simulink library "libAggregators"  (R2015a)
settings: Solver=ode45  StartTime=0.0  StopTime=10.0  RelTol=1e-3
libraries: dspsigattribs x4, libAggregators x1
settings Model: Creator=jcardena  LastModifiedBy=jcardena
settings DebuggingCC: UnderspecifiedInitializationDetection=Classic  MergeDetectMultiDrivingBlocksExec=none  SolverPrmCheckMsg=warning  StateNameClashWarn=warning

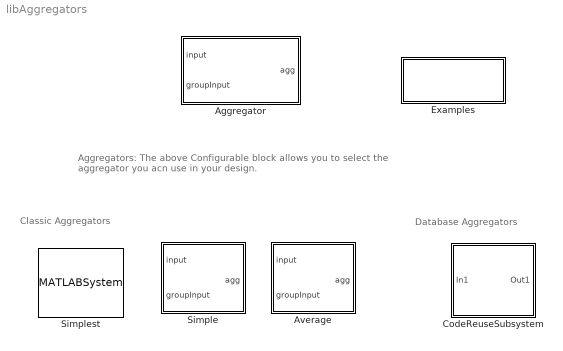
== system libAggregators ==
  note: Aggregators: The above Configurable block allows you to select the aggregator you acn use in your design.
  note: Database Aggregators
  note: Classic Aggregators
  Aggregator : Subsystem  BlockChoice=Average
      settings: TemplateBlock=self  MemberBlocks=Average,Simple
  Average : Subsystem  mask(aggregatingBlock){gVal=1}
      mask prompts: gVal "Grouping expression or value"
      mask help: An Aggregator classifies data rows from a single input link into groups and computes totals or other aggregate functions for each group. The averaged totals for each group are output from the stage via an output port.
      settings: RTWFcnNameOpts=Use subsystem name  RTWFileNameOpts=Use function name
      mask Help: Enter the aggregate function
      mask Display: image('images/aggrIcon.png')
  CodeReuseSubsystem : Subsystem  TreatAsAtomicUnit=on  mask(Aggregator Type){}
      mask help: Aggregator description
      settings: RTWFcnNameOpts=Use subsystem name  RTWFileNameOpts=Use function name
  Examples : Subsystem  mask(Aggregator Examples){}
      mask Display: disp('Aggregator\nExamples')
  Simple : Subsystem  mask(aggregatingBlock){gVal=1}
      mask prompts: gVal "Grouping expression or value"
      mask help: An Aggregator classifies data rows from a single input link into groups and computes totals or other aggregate functions for each group. The summed totals for each group are output from the stage via an output port.
      mask Help: Enter the aggregate function
      mask Display: image('images/aggrIcon.png')
  Simplest : MATLABSystem  System=simplestAggregator_mtlbSysBlock
      mask Type: simplestAggregator_mtlbSysBlock
      mask Display:
      | disp('Simplest');
      | port_label('output',1,'agg');

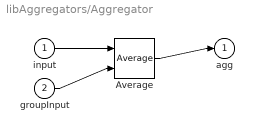
== system libAggregators/Aggregator ==
  input : Inport
  groupInput : Inport  Port=2
  Average : libAggregators/Average  gVal=1
  agg : Outport
  wires:
  input/1 -> Average/1
  groupInput/1 -> Average/2
  Average/1 -> agg/1

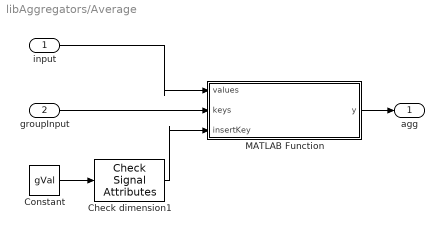
== system libAggregators/Average ==
  input : Inport
  groupInput : Inport  Port=2
  Check dimension1 : dspsigattribs/Check Signal Attributes  SigAttribCheckMethod=Does not match attributes exactly  Complexity=Ignore  Frame=Ignore  DimsCheckMethod=Is...  Dimensions=Vector (1-D or 2-D)  DatatypeCheckMethod=Ignore  DatatypeGeneral=Floating-point  DtypeFloatSpecific=Any floating-point  DtypeFixedSpecific=Any fixed-point  DtypeIntSpecific=Any integer  SampleMode=Ignore
  Constant : Constant  Value=gVal
  MATLAB Function : MATLAB Function  TreatAsAtomicUnit=on
      settings: RTWSystemCode=Inline
  agg : Outport
  wires:
  input/1 -> MATLAB Function/1(values)
  groupInput/1 -> MATLAB Function/2(keys)
  Constant/1 -> Check dimension1/1
  MATLAB Function/1(y) -> agg/1
  Check dimension1/1 -> MATLAB Function/3(insertKey)

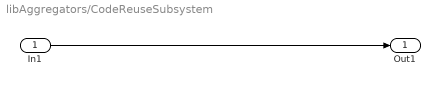
== system libAggregators/CodeReuseSubsystem ==
  In1 : Inport
  Out1 : Outport
  wires:
  In1/1 -> Out1/1

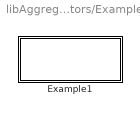
== system libAggregators/Examples ==
  Example1 : Subsystem
      settings: OpenFcn=read_simulated_unitIDs_example

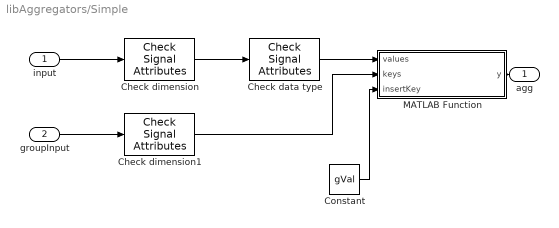
== system libAggregators/Simple ==
  input : Inport
  groupInput : Inport  Port=2
  Check data type : dspsigattribs/Check Signal Attributes  SigAttribCheckMethod=Does not match attributes exactly  Complexity=Ignore  Frame=Ignore  DimsCheckMethod=Ignore  Dimensions=Full matrix (2-D)  DatatypeCheckMethod=Is...  DatatypeGeneral=Floating-point  DtypeFloatSpecific=Double precision  DtypeFixedSpecific=Any fixed-point  DtypeIntSpecific=Any integer  SampleMode=Ignore
  Check dimension : dspsigattribs/Check Signal Attributes  SigAttribCheckMethod=Does not match attributes exactly  Complexity=Ignore  Frame=Ignore  DimsCheckMethod=Is...  Dimensions=Vector (1-D or 2-D)  DatatypeCheckMethod=Ignore  DatatypeGeneral=Floating-point  DtypeFloatSpecific=Any floating-point  DtypeFixedSpecific=Any fixed-point  DtypeIntSpecific=Any integer  SampleMode=Ignore
  Check dimension1 : dspsigattribs/Check Signal Attributes  SigAttribCheckMethod=Does not match attributes exactly  Complexity=Ignore  Frame=Ignore  DimsCheckMethod=Is...  Dimensions=Vector (1-D or 2-D)  DatatypeCheckMethod=Ignore  DatatypeGeneral=Floating-point  DtypeFloatSpecific=Any floating-point  DtypeFixedSpecific=Any fixed-point  DtypeIntSpecific=Any integer  SampleMode=Ignore
  Constant : Constant  Value=gVal
  MATLAB Function : MATLAB Function  TreatAsAtomicUnit=on
      settings: RTWSystemCode=Inline
  agg : Outport
  wires:
  groupInput/1 -> Check dimension1/1
  Check dimension/1 -> Check data type/1
  input/1 -> Check dimension/1
  Check dimension1/1 -> MATLAB Function/2(keys)
  MATLAB Function/1(y) -> agg/1
  Check data type/1 -> MATLAB Function/1(values)
  Constant/1 -> MATLAB Function/3(insertKey)

== system libAggregators/Examples/Example1 ==

== matlab function libAggregators/Average/MATLAB Function ==
  data: values input; y output; keys input; insertKey input
function y = avgAggr(values, keys, insertKey)
%#codegen
index = keys == insertKey;
y = mean(values(index));

== matlab function libAggregators/Simple/MATLAB Function ==
  data: values input; y output; keys input; insertKey input
function y = sumAggr(values, keys, insertKey)
%#codegen
index = keys == insertKey;
y = sum(values(index));
